simulink model "allInOne"  (R2018b)
settings: Solver=FixedStepDiscrete  StartTime=0.0  StopTime=inf  FixedStep=1/50  RelTol=1e-3  EnableMultiTasking=on
PreLoadFcn:
  | BOD_startup
  | BOW_startup
values from neighbouring files (symbols this model uses):
  K = Kext(1:6)    [BOW_startup.m]
  Rp = 4e-3    (= 0.004)    [BOW_startup.m]
undefined symbols (not defined in the file or in its folder): Ad, Ad1, Bd, Bd1, C, Cd, Dfilter, DiscIntNeverNeededParam, Discrete, F, G, K1, K2, K3, Kd, Ki, KN, Kp, KR, P_const, P_offset, sat, Time
libraries: simulink x4, ctrlSharedLib x4, embdlinuxlib x2
settings Model: SimulationMode=external  Creator=Josef  LastModifiedBy=Adam
settings SolverCC: PositivePriorityOrder=on
settings OptimizationCC: PassReuseOutputArgsThreshold=0  MaxStackSize=64
settings DebuggingCC: ParameterTunabilityLossMsg=error
settings HardwareCC: ProdBitPerPointer=32  ProdBitPerSizeT=32  ProdBitPerPtrDiffT=32  ProdLargestAtomicInteger=Long  ProdLargestAtomicFloat=Double  ProdWordSize=32  ProdHWDeviceType=ARM Compatible->ARM Cortex  UseEmbeddedCoderFeatures=off
settings SFSimCC: SimUseLocalCustomCode=off  MATLABDynamicMemAlloc=off
settings RTWCC: SystemTargetFile=ert.tlc  HardwareBoard=Raspberry Pi  TLCOptions="-aInlineSetEventsForThisBaseRateFcn=TLC_FALSE -aSuppressMultiTaskScheduler=TLC_FALSE  -aRateBasedStepFcn=0"  TemplateMakefile=ert_default_tmf  GenerateReport=on  RTWUseLocalCustomCode=off  Toolchain=GNU GCC Raspberry Pi  TargetLang=C++
settings CodeAppCC: ForceParamTrailComments=on  OperatorAnnotations=on  StateflowObjectComments=on
settings ERTTargetCC: TargetLangStandard=C++03 (ISO)  ERTCustomFileBanners=off  SupportContinuousTime=on  SupportNonInlinedSFcns=on  RemoveResetFunc=off  SupportVariableSizeSignals=on  ModelStepFunctionPrototypeControlCompliant=off

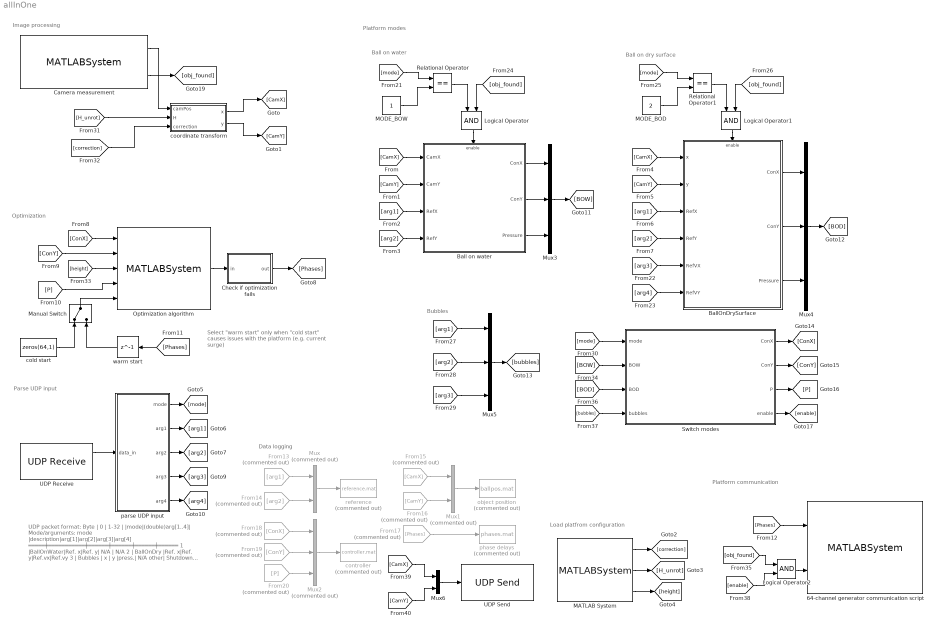
== system allInOne ==
  note: Platform modes
  note: UDP packet format:
      | Byte | 0 | 1-32 |
      | |mode|(double)arg[1..4]|
      |
      | Mode/arguments:
      | mode |description|arg[1]|arg[2]|arg[3]|arg[4]
      | ═════╪═══════════╪══════╪══════╪══════╪══════
      | 1 |BallOnWater|Ref. x|Ref. y| N/A | N/A
      | 2 | BallOnDry |Ref. x|Ref. y|Ref.vx|Ref.vy
      | 3 | Bubbles | x | y |press.| N/A
      | other| Shutdown | N/A | N/A | N/A | N/A
  note: Load platfrom configuration
  note: Select "warm start" only when
      | "cold start" causes issues with
      | the platform (e.g. current surge)
  note: Data logging
  note: Parse UDP input
  note: Platform communication
  note: Optimization
  note: Image processing
  note: Bubbles
  note: Ball on dry surface
  note: Ball on water
  64-channel generator communication script : MATLABSystem  System=NewGenerator  Port=/dev/ttyUSB0  Baud=230400
      mask Type: NewGenerator
      mask Display:
      | disp(['64 phase generator' char(10) ' Port: /dev/ttyUSB0' char(10) ' Baudrate: 230400']);
      | port_label('input',1,'phases');
      | port_label('input',2,'On/Off');
  Ball on water : Subsystem
  BallOnDrySurface : Subsystem
  Camera measurement : MATLABSystem  System=RaspiBallPos  shm_key=3145914  framerate=50  N=1000  objects=1  km=eye( 3 )  notfound=0  execScript=off  concatenateOutputs=off  rotation=off  found_output=on
      mask Type: RaspiBallPos
      mask Display:
      | disp('RaspiBallPos');
      | port_label('output',1,'Position 1 [x;y]');
      | port_label('output',2,'Object found?');
  Check if optimization fails : MATLAB Function  TreatAsAtomicUnit=on
  From13 : From  Commented=on  GotoTag=arg1
  From14 : From  Commented=on  GotoTag=arg2
  From15 : From  Commented=on  GotoTag=CamX
  From16 : From  Commented=on  GotoTag=CamY
  From17 : From  Commented=on  GotoTag=Phases
  From18 : From  Commented=on  GotoTag=ConX
  From19 : From  Commented=on  GotoTag=ConY
  From20 : From  Commented=on  GotoTag=P
  Logical Operator : Logic  AllPortsSameDT=off  OutDataTypeStr=boolean
  Logical Operator1 : Logic  AllPortsSameDT=off  OutDataTypeStr=boolean
  Logical Operator2 : Logic  AllPortsSameDT=off  OutDataTypeStr=boolean
  MATLAB System : MATLABSystem  System=Loader  corrFile=/home/pi/correction.bin  H_unFile=/home/pi/H_unrot.bin  heightFile=/home/pi/height.bin
      mask Type: Loader
      mask Display:
      | disp('Loader');
      | port_label('output',1,'correction');
      | port_label('output',2,'H_unrot');
      | port_label('output',3,'height');
  "MODE_BOD " : Constant  Value=2
  MODE_BOW : Constant
  Manual Switch : ManualSwitch
  Mux : Mux  Commented=on  Inputs=2
  Mux1 : Mux  Commented=on  Inputs=2
  Mux2 : Mux  Commented=on  Inputs=3
  Mux3 : Mux  Inputs=3
  Mux4 : Mux  Inputs=3
  Mux5 : Mux  Inputs=3
  Mux6 : Mux  Inputs=2
  Optimization algorithm : MATLABSystem  System=PressurePoints
      mask Type: PressurePoints
      mask Display:
      | disp(['Pressure points' char(10) 'optimization']);
      | port_label('input',1,'x');
      | port_label('input',2,'y');
      | port_label('input',3,'z');
      | port_label('input',4,'Required pressure');
      | port_label('input',5,'Initial condition');
      | port_label('output',1,'Phases');
  Relational Operator : RelationalOperator  Operator===  OutDataTypeStr=boolean  RndMeth=Simplest
  Relational Operator1 : RelationalOperator  Operator===  OutDataTypeStr=boolean  RndMeth=Simplest
  Switch modes : MATLAB Function  TreatAsAtomicUnit=on
  UDP Receive : embdlinuxlib/UDP Receive  localURL='0.0.0.0'  localPort=25000  remoteURL='0.0.0.0'  remotePort=-1  recvBufferSize=8192  signalDatatype=uint8  dims=33  isVarSize=off  showBlockingTime=off  blockingTime=0  sampletime=1/50  blockPlatform=Raspberry Pi
      settings: SourceProductName=Simulink Support Package for Raspberry Pi Hardware  SourceProductBaseCode=RASPPI
  UDP Send : embdlinuxlib/UDP Send  remoteURL='127.0.0.1'  remotePort=25001  localURL='255.255.255.255'  localPortSource=Automatically determine  localPort=-1  sampletime=-1  blockPlatform=Raspberry Pi  separateLengthPort=0
      settings: SourceProductName=Simulink Support Package for Raspberry Pi Hardware  SourceProductBaseCode=RASPPI
  cold start : Constant  Value=zeros(64,1)
  controller : ToFile  Commented=on  Filename=controller.mat  MatrixName=controller
  coordinate transform : MATLAB Function  TreatAsAtomicUnit=on
  object position : ToFile  Commented=on  Filename=ballpos.mat  MatrixName=ballpos
  parse UDP input : MATLAB Function  TreatAsAtomicUnit=on
  phase delays : ToFile  Commented=on  Filename=phases.mat  MatrixName=phases
  reference : ToFile  Commented=on  Filename=reference.mat  MatrixName=ref
  warm start : Delay  DelayLength=1  InitialCondition=zeros(64,1)
  wires:
  coordinate transform/1(x) -> [CamX]
  [H_unrot] -> coordinate transform/2(H)
  coordinate transform/2(y) -> [CamY]
  Camera measurement/1 -> coordinate transform/1(camPos)
  [correction] -> coordinate transform/3(correction)
  Check if optimization fails/1(out) -> [Phases]
  [ConX] -> Optimization algorithm/1
  [ConY] -> Optimization algorithm/2
  [Phases] -> warm start/1
  [P] -> Optimization algorithm/4
  Optimization algorithm/1 -> Check if optimization fails/1(in)
  cold start/1 -> Manual Switch/1
  warm start/1 -> Manual Switch/2
  Manual Switch/1 -> Optimization algorithm/5
  [height] -> Optimization algorithm/3
  [Phases] -> 64-channel generator communication script/1
  [obj_found] -> Logical Operator2/1
  From13/1 -> Mux/1
  From15/1 -> Mux1/1
  Mux1/1 -> object position/1
  From16/1 -> Mux1/2
  From18/1 -> Mux2/1
  From20/1 -> Mux2/3
  From19/1 -> Mux2/2
  Mux/1 -> reference/1
  From14/1 -> Mux/2
  From17/1 -> phase delays/1
  Mux2/1 -> controller/1
  MATLAB System/3 -> [height]
  MATLAB System/2 -> [H_unrot]
  MATLAB System/1 -> [correction]
  Camera measurement/2 -> [obj_found]
  UDP Receive/1 -> parse UDP input/1(data_in)
  parse UDP input/1(mode) -> [mode]
  parse UDP input/2(arg1) -> [arg1]
  parse UDP input/3(arg2) -> [arg2]
  parse UDP input/4(arg3) -> [arg3]
  parse UDP input/5(arg4) -> [arg4]
  [CamX] -> BallOnDrySurface/1(x)
  [arg1] -> BallOnDrySurface/3(RefX)
  Relational Operator/1 -> Logical Operator/1
  [arg2] -> BallOnDrySurface/4(RefY)
  [arg3] -> BallOnDrySurface/5(RefVX)
  MODE_BOW/1 -> Relational Operator/2
  Ball on water/2(ConY) -> Mux3/2
  [BOD] -> Switch modes/3(BOD)
  [CamY] -> BallOnDrySurface/2(y)
  [arg4] -> BallOnDrySurface/6(RefVY)
  BallOnDrySurface/2(ConY) -> Mux4/2
  BallOnDrySurface/1(ConX) -> Mux4/1
  [arg1] -> Mux5/1
  [arg2] -> Mux5/2
  [mode] -> Relational Operator/1
  BallOnDrySurface/3(Pressure) -> Mux4/3
  Mux5/1 -> [bubbles]
  Switch modes/3(P) -> [P]
  Ball on water/3(Pressure) -> Mux3/3
  [mode] -> Switch modes/1(mode)
  [CamY] -> Ball on water/2(CamY)
  Logical Operator/1 -> Ball on water/Enable
  "MODE_BOD "/1 -> Relational Operator1/2
  [mode] -> Relational Operator1/1
  [obj_found] -> Logical Operator1/2
  Logical Operator1/1 -> BallOnDrySurface/Enable
  Relational Operator1/1 -> Logical Operator1/1
  Mux3/1 -> [BOW]
  Switch modes/4(enable) -> [enable]
  Ball on water/1(ConX) -> Mux3/1
  [CamX] -> Ball on water/1(CamX)
  [arg2] -> Ball on water/4(RefY)
  [BOW] -> Switch modes/2(BOW)
  [arg1] -> Ball on water/3(RefX)
  [obj_found] -> Logical Operator/2
  [bubbles] -> Switch modes/4(bubbles)
  [arg3] -> Mux5/3
  Switch modes/1(ConX) -> [ConX]
  Switch modes/2(ConY) -> [ConY]
  Mux4/1 -> [BOD]
  Logical Operator2/1 -> 64-channel generator communication script/2
  [enable] -> Logical Operator2/2
  Mux6/1 -> UDP Send/1
  [CamX] -> Mux6/1
  [CamY] -> Mux6/2

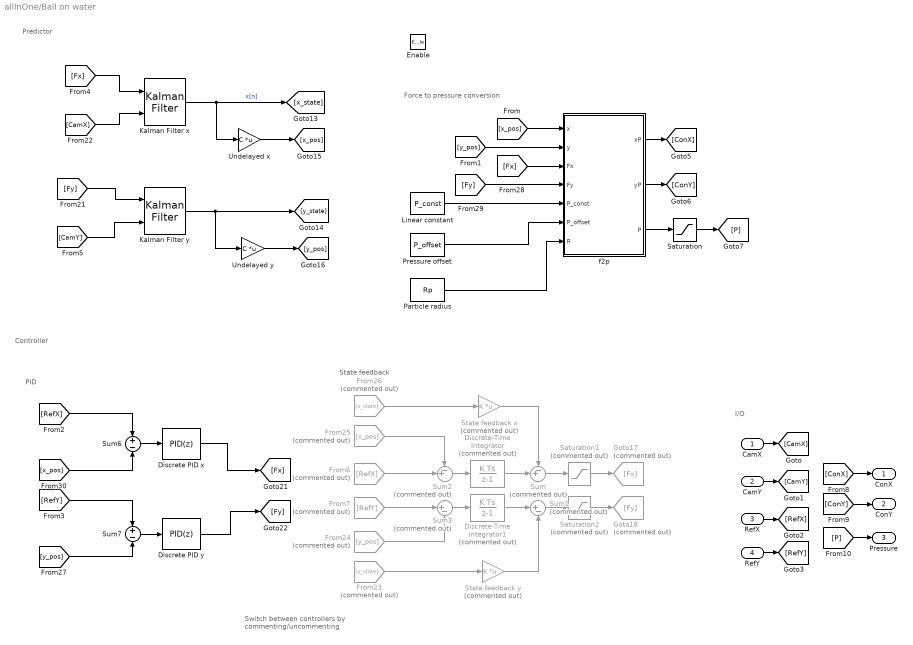
== system allInOne/Ball on water ==
  note: I/O
  note: Force to pressure conversion
  note: PID
  note: State feedback
  note: Switch between controllers by
      | commenting/uncommenting
  note: Controller
  note: Predictor
  CamX : Inport
  CamY : Inport  Port=2
  RefX : Inport  Port=3
  RefY : Inport  Port=4
  Enable : EnablePort  StatesWhenEnabling=reset
  Discrete PID x : simulink/Continuous/PID Controller  Controller=PID  Form=Parallel  TimeDomain=Discrete-time  SampleTime=-1  IntegratorMethod=Forward Euler  FilterMethod=Forward Euler  ControllerParametersSource=internal  P=Kp  I=Ki  D=Kd  UseFilter=on  N=Dfilter  TunerSelectOption=Transfer Function Based (PID Tuner App)  InitialConditionSource=internal  InitialConditionForIntegrator=0  InitialConditionForFilter=0  DifferentiatorICPrevScaledInput=0  ExternalReset=none  TrackingMode=off  Kt=1  LimitOutput=on  UpperSaturationLimit=sat  LowerSaturationLimit=-sat  LinearizeAsGain=off  AntiWindupMode=clamping  Kb=1  POutMin=[]  POutMax=[]  IOutMin=[]  IOutMax=[]  DOutMin=[]  DOutMax=[]  NOutMin=[]  NOutMax=[]  SumOutMin=[]  SumOutMax=[]  SaturationOutMin=[]  SaturationOutMax=[]  PParamMin=[]  PParamMax=[]  IParamMin=[]  IParamMax=[]  DParamMin=[]  DParamMax=[]  NParamMin=[]  NParamMax=[]  KbParamMin=[]  KbParamMax=[]  KtParamMin=[]  KtParamMax=[]  KbOutMin=[]  KbOutMax=[]  KtOutMin=[]  KtOutMax=[]  IntegratorOutMin=[]  IntegratorOutMax=[]  FilterOutMin=[]  FilterOutMax=[]  SumI1OutMin=[]  SumI1OutMax=[]  SumI2OutMin=[]  SumI2OutMax=[]  SumI3OutMin=[]  SumI3OutMax=[]  SumI4OutMin=[]  SumI4OutMax=[]  SumDOutMin=[]  SumDOutMax=[]  DifferentiatorOutMin=[]  DifferentiatorOutMax=[]  FilterDiffOutCoefMin=[]  FilterDiffOutCoefMax=[]  ReciprocalOutMin=[]  ReciprocalOutMax=[]  SumDenOutMin=[]  SumDenOutMax=[]  SumNumOutMin=[]  SumNumOutMax=[]  DivideOutMin=[]  DivideOutMax=[]  IntegratorContinuousStateAttributes=''  IntegratorStateMustResolveToSignalObject=off  IntegratorRTWStateStorageClass=Auto  FilterContinuousStateAttributes=''  FilterStateMustResolveToSignalObject=off  FilterRTWStateStorageClass=Auto  ParallelPVariant=InternalParameters  IdealPVariant=Disabled  IVariant=InternalParameters  DVariant=InternalParameters  IntegratorVariant=Discrete  SatVariant=Enabled  AWVariant=DiscClampingParallel  PCopyVariant=Disabled  TRVariant=Disabled  FdbkBlocksVariant=Forward  IdealPFdbkVariant=Disabled  SatFdbkVariant=Disabled  DerivativeFilterVariant=ForwardEulerFilter  NVariant=InternalParameters  NCopyVariant=Disabled  FilterICVariant=InternalICsFilter  IntegratorICVariant=InternalICs  ExternalResetVariant=Disabled  TRSumVariant=Passthrough  SumFdbkVariant=Disabled  SumVariant=Sum_PID
  Discrete PID y : simulink/Continuous/PID Controller  Controller=PID  Form=Parallel  TimeDomain=Discrete-time  SampleTime=-1  IntegratorMethod=Forward Euler  FilterMethod=Forward Euler  ControllerParametersSource=internal  P=Kp  I=Ki  D=Kd  UseFilter=on  N=Dfilter  TunerSelectOption=Frequency Response Based  InitialConditionSource=internal  InitialConditionForIntegrator=0  InitialConditionForFilter=0  DifferentiatorICPrevScaledInput=0  ExternalReset=none  TrackingMode=off  Kt=1  LimitOutput=on  UpperSaturationLimit=sat  LowerSaturationLimit=-sat  LinearizeAsGain=off  AntiWindupMode=clamping  Kb=1  POutMin=[]  POutMax=[]  IOutMin=[]  IOutMax=[]  DOutMin=[]  DOutMax=[]  NOutMin=[]  NOutMax=[]  SumOutMin=[]  SumOutMax=[]  SaturationOutMin=[]  SaturationOutMax=[]  PParamMin=[]  PParamMax=[]  IParamMin=[]  IParamMax=[]  DParamMin=[]  DParamMax=[]  NParamMin=[]  NParamMax=[]  KbParamMin=[]  KbParamMax=[]  KtParamMin=[]  KtParamMax=[]  KbOutMin=[]  KbOutMax=[]  KtOutMin=[]  KtOutMax=[]  IntegratorOutMin=[]  IntegratorOutMax=[]  FilterOutMin=[]  FilterOutMax=[]  SumI1OutMin=[]  SumI1OutMax=[]  SumI2OutMin=[]  SumI2OutMax=[]  SumI3OutMin=[]  SumI3OutMax=[]  SumI4OutMin=[]  SumI4OutMax=[]  SumDOutMin=[]  SumDOutMax=[]  DifferentiatorOutMin=[]  DifferentiatorOutMax=[]  FilterDiffOutCoefMin=[]  FilterDiffOutCoefMax=[]  ReciprocalOutMin=[]  ReciprocalOutMax=[]  SumDenOutMin=[]  SumDenOutMax=[]  SumNumOutMin=[]  SumNumOutMax=[]  DivideOutMin=[]  DivideOutMax=[]  IntegratorContinuousStateAttributes=''  IntegratorStateMustResolveToSignalObject=off  IntegratorRTWStateStorageClass=Auto  FilterContinuousStateAttributes=''  FilterStateMustResolveToSignalObject=off  FilterRTWStateStorageClass=Auto  ParallelPVariant=InternalParameters  IdealPVariant=Disabled  IVariant=InternalParameters  DVariant=InternalParameters  IntegratorVariant=Discrete  SatVariant=Enabled  AWVariant=DiscClampingParallel  PCopyVariant=Disabled  TRVariant=Disabled  FdbkBlocksVariant=Forward  IdealPFdbkVariant=Disabled  SatFdbkVariant=Disabled  DerivativeFilterVariant=ForwardEulerFilter  NVariant=InternalParameters  NCopyVariant=Disabled  FilterICVariant=InternalICsFilter  IntegratorICVariant=InternalICs  ExternalResetVariant=Disabled  TRSumVariant=Passthrough  SumFdbkVariant=Disabled  SumVariant=Sum_PID
  Discrete-Time Integrator : DiscreteIntegrator  Commented=on  gainval=K_i  SampleTime=1/50  UpperSaturationLimit=sat  LowerSaturationLimit=-sat  ICPrevOutput=DiscIntNeverNeededParam  ICPrevScaledInput=DiscIntNeverNeededParam
  Discrete-Time Integrator1 : DiscreteIntegrator  Commented=on  gainval=K_i  SampleTime=1/50  UpperSaturationLimit=sat  LowerSaturationLimit=-sat  ICPrevOutput=DiscIntNeverNeededParam  ICPrevScaledInput=DiscIntNeverNeededParam
  From23 : From  Commented=on  GotoTag=y_state
  From24 : From  Commented=on  GotoTag=y_pos
  From25 : From  Commented=on  GotoTag=x_pos
  From26 : From  Commented=on  GotoTag=x_state
  From6 : From  Commented=on  GotoTag=RefX
  From7 : From  Commented=on  GotoTag=RefY
  Goto17 : Goto  Commented=on  GotoTag=Fx
  Goto18 : Goto  Commented=on  GotoTag=Fy
  Kalman Filter x : ctrlSharedLib/Kalman Filter  TimeDomain=Discrete-Time  UseCurrentEstimator=on  ModelSource=Individual A, B, C, D matrices  ModelSourceVariable=ss(0.95,1,1,0,1)  A=F  B=G  C=C  D=0  NumberOfStates=1  NumberOfInputs=1  NumberOfOutputs=1  InitialEstimateSource=Dialog  X0=0  P0=10  UseK=off  UseGH=off  NumberOfProcessNoiseInputs=1  G=1  TimeInvariantG=on  H=0  TimeInvariantH=on  Q=KQ  TimeInvariantQ=on  R=KR  TimeInvariantR=on  N=KN  TimeInvariantN=on  AddInputPort=on  AddEnablePort=off  OutputEstimatedY=off  OutputP=off  Ts=1/50
      settings: SourceProductBaseCode=CT
  Kalman Filter y : ctrlSharedLib/Kalman Filter  TimeDomain=Discrete-Time  UseCurrentEstimator=on  ModelSource=Individual A, B, C, D matrices  ModelSourceVariable=ss(0.95,1,1,0,1)  A=F  B=G  C=C  D=0  NumberOfStates=1  NumberOfInputs=1  NumberOfOutputs=1  InitialEstimateSource=Dialog  X0=0  P0=10  UseK=off  UseGH=off  NumberOfProcessNoiseInputs=1  G=1  TimeInvariantG=on  H=0  TimeInvariantH=on  Q=KQ  TimeInvariantQ=on  R=KR  TimeInvariantR=on  N=KN  TimeInvariantN=on  AddInputPort=on  AddEnablePort=off  OutputEstimatedY=off  OutputP=off  Ts=1/50
      settings: SourceProductBaseCode=CT
  Linear constant : Constant  Value=P_const
  Particle radius : Constant  Value=Rp
  Pressure offset : Constant  Value=P_offset
  Saturation : Saturate  UpperLimit=2500  LowerLimit=0
  Saturation1 : Saturate  Commented=on  UpperLimit=sat  LowerLimit=-sat
  Saturation2 : Saturate  Commented=on  UpperLimit=sat  LowerLimit=-sat
  State feedback x : Gain  Commented=on  Gain=K  Multiplication=Matrix(K*u) (u vector)
  State feedback y : Gain  Commented=on  Gain=K  Multiplication=Matrix(K*u) (u vector)
  Sum : Sum  Commented=on  Inputs=-+|
  Sum1 : Sum  Commented=on  Inputs=|+-
  Sum2 : Sum  Commented=on  Inputs=-+|
  Sum3 : Sum  Commented=on  Inputs=|+-
  Sum6 : Sum  Inputs=+-
  Sum7 : Sum  Inputs=+-
  Undelayed x : Gain  Gain=C  Multiplication=Matrix(K*u)
  Undelayed y : Gain  Gain=C  Multiplication=Matrix(K*u)
  f2p : MATLAB Function  TreatAsAtomicUnit=on
  ConX : Outport
  ConY : Outport  Port=2
  Pressure : Outport  Port=3
  wires:
  [Fx] -> f2p/3(Fx)
  Pressure offset/1 -> f2p/6(P_offset)
  [x_pos] -> f2p/1(x)
  f2p/2(yP) -> [ConY]
  [Fy] -> f2p/4(Fy)
  Linear constant/1 -> f2p/5(P_const)
  Discrete PID x/1 -> [Fx]
  Discrete PID y/1 -> [Fy]
  f2p/3(P) -> Saturation/1
  [y_pos] -> f2p/2(y)
  Undelayed y/1 -> [y_pos]
  f2p/1(xP) -> [ConX]
  Saturation/1 -> [P]
  Particle radius/1 -> f2p/7(R)
  Undelayed x/1 -> [x_pos]
  Saturation2/1 -> Goto18/1
  Saturation1/1 -> Goto17/1
  Sum7/1 -> Discrete PID y/1
  [RefY] -> Sum7/1
  [y_pos] -> Sum7/2
  [x_pos] -> Sum6/2
  Sum6/1 -> Discrete PID x/1
  [RefX] -> Sum6/1
  [CamX] -> Kalman Filter x/2
  [Fx] -> Kalman Filter x/1
  Sum/1 -> Saturation1/1
  From26/1 -> State feedback x/1
  From7/1 -> Sum3/1
  From23/1 -> State feedback y/1
  From25/1 -> Sum2/1
  Sum1/1 -> Saturation2/1
  From24/1 -> Sum3/2
  From6/1 -> Sum2/2
  Sum3/1 -> Discrete-Time Integrator1/1
  State feedback x/1 -> Sum/1
  Sum2/1 -> Discrete-Time Integrator/1
  Discrete-Time Integrator/1 -> Sum/2
  Discrete-Time Integrator1/1 -> Sum1/1
  State feedback y/1 -> Sum1/2
  [ConX] -> ConX/1
  [ConY] -> ConY/1
  [P] -> Pressure/1
  CamX/1 -> [CamX]
  RefX/1 -> [RefX]
  CamY/1 -> [CamY]
  RefY/1 -> [RefY]
  [Fy] -> Kalman Filter y/1
  [CamY] -> Kalman Filter y/2
  Kalman Filter x/1 -> Undelayed x/1, [x_state]  "x[n]"
  Kalman Filter y/1 -> Undelayed y/1, [y_state]

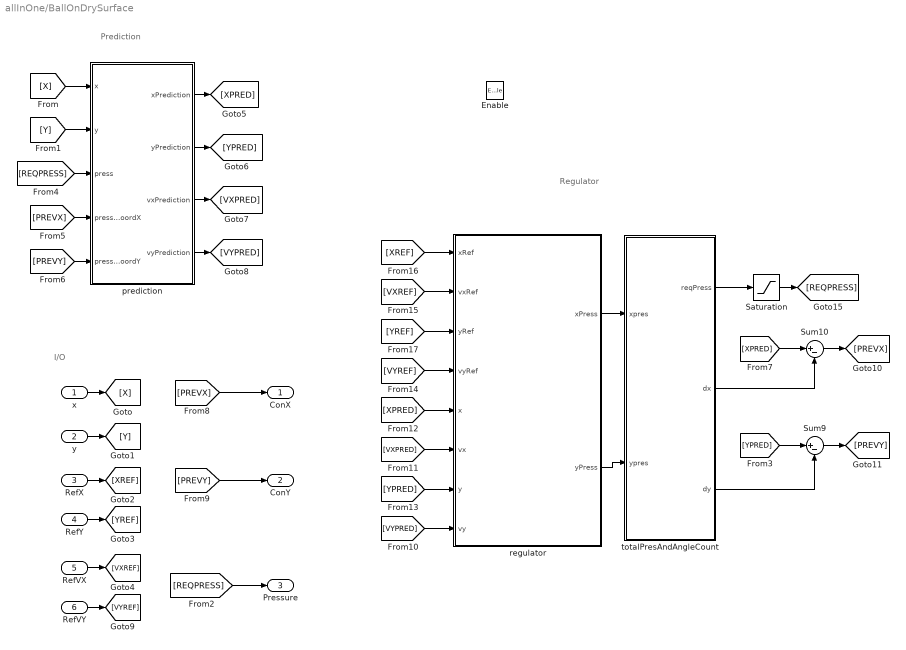
== system allInOne/BallOnDrySurface ==
  note: Prediction
  note: Regulator
  note: I/O
  x : Inport
  y : Inport  Port=2
  RefX : Inport  Port=3
  RefY : Inport  Port=4
  RefVX : Inport  Port=5
  RefVY : Inport  Port=6
  Enable : EnablePort  StatesWhenEnabling=reset
  Saturation : Saturate  UpperLimit=3300  LowerLimit=0
  Sum10 : Sum  Inputs=|+-
  Sum9 : Sum  Inputs=|+-
  prediction : Subsystem
  "regulator " : Subsystem
  totalPresAndAngleCount : MATLAB Function  TreatAsAtomicUnit=on
  ConX : Outport
  ConY : Outport  Port=2
  Pressure : Outport  Port=3
  wires:
  [X] -> prediction/1(x)
  prediction/4(vyPrediction) -> [VYPRED]
  prediction/3("vxPrediction ") -> [VXPRED]
  [REQPRESS] -> prediction/3("press ")
  [Y] -> prediction/2(y)
  prediction/2(yPrediction) -> [YPRED]
  prediction/1(xPrediction) -> [XPRED]
  [PREVY] -> prediction/5("pressCoordY ")
  [PREVX] -> prediction/4(pressCoordX)
  [XPRED] -> "regulator "/5(x)
  [VXREF] -> "regulator "/2(vxRef)
  [VXPRED] -> "regulator "/6(vx)
  [YPRED] -> "regulator "/7(y)
  [XREF] -> "regulator "/1(xRef)
  Saturation/1 -> [REQPRESS]
  [YREF] -> "regulator "/3(yRef)
  "regulator "/2(yPress) -> totalPresAndAngleCount/2(ypres)
  "regulator "/1(xPress) -> totalPresAndAngleCount/1(xpres)
  totalPresAndAngleCount/1(reqPress) -> Saturation/1
  [VYREF] -> "regulator "/4(vyRef)
  [VYPRED] -> "regulator "/8(vy)
  x/1 -> [X]
  Sum10/1 -> [PREVX]
  y/1 -> [Y]
  RefX/1 -> [XREF]
  Sum9/1 -> [PREVY]
  RefY/1 -> [YREF]
  [REQPRESS] -> Pressure/1
  RefVY/1 -> [VYREF]
  RefVX/1 -> [VXREF]
  [YPRED] -> Sum9/1
  [XPRED] -> Sum10/1
  totalPresAndAngleCount/2(dx) -> Sum10/2
  totalPresAndAngleCount/3(dy) -> Sum9/2
  [PREVX] -> ConX/1
  [PREVY] -> ConY/1

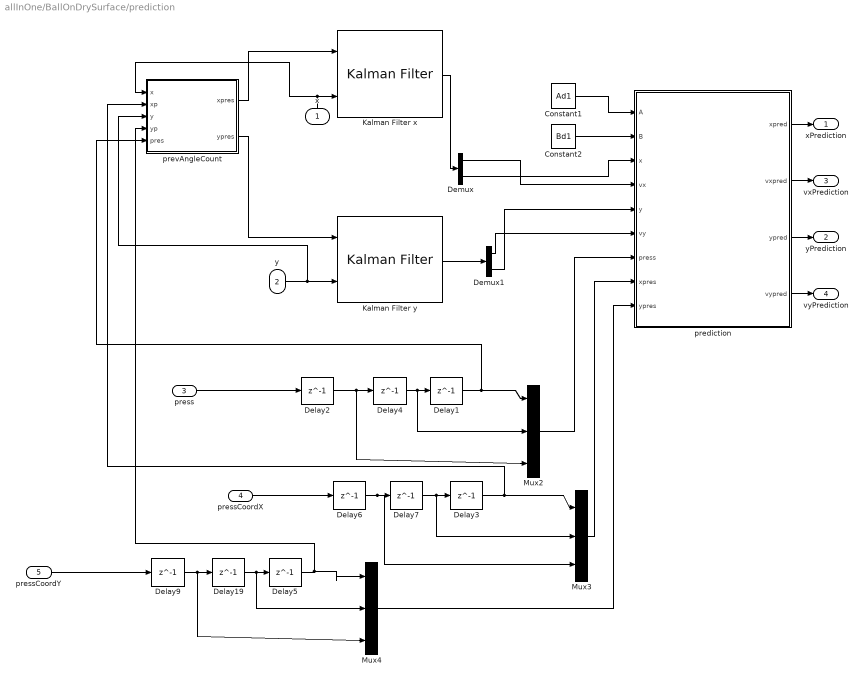
== system allInOne/BallOnDrySurface/prediction ==
  x : Inport  SampleTime=1/50
  y : Inport  Port=2  SampleTime=1/50
  "press " : Inport  Port=3
  pressCoordX : Inport  Port=4
  "pressCoordY " : Inport  Port=5
  Constant1 : Constant  Value=Ad1  SampleTime=-1
  Constant2 : Constant  Value=Bd1  SampleTime=-1
  Delay{1..7,9,19} (9 alike) : Delay  DelayLength=1
  Demux : Demux  Outputs=2
  Demux1 : Demux  Outputs=2
  Kalman Filter x : ctrlSharedLib/Kalman Filter  TimeDomain=Discrete-Time  UseCurrentEstimator=on  ModelSource=Individual A, B, C, D matrices  ModelSourceVariable=ss(0.95,1,1,0,1)  A=Ad  B=Bd  C=Cd  D=0  NumberOfStates=1  NumberOfInputs=1  NumberOfOutputs=1  InitialEstimateSource=Dialog  X0=[0;0]  P0=10  UseK=off  UseGH=off  NumberOfProcessNoiseInputs=1  G=1  TimeInvariantG=on  H=0  TimeInvariantH=on  Q=[5e-5 0 ; 0 1e-7]  TimeInvariantQ=on  R=7e-12;  TimeInvariantR=on  N=0  TimeInvariantN=on  AddInputPort=on  AddEnablePort=off  OutputEstimatedY=off  OutputP=off  Ts=-1
      settings: SourceProductBaseCode=CT
  Kalman Filter y : ctrlSharedLib/Kalman Filter  TimeDomain=Discrete-Time  UseCurrentEstimator=on  ModelSource=Individual A, B, C, D matrices  ModelSourceVariable=ss(0.95,1,1,0,1)  A=Ad  B=Bd  C=Cd  D=0  NumberOfStates=1  NumberOfInputs=1  NumberOfOutputs=1  InitialEstimateSource=Dialog  X0=[0;0]  P0=10  UseK=off  UseGH=off  NumberOfProcessNoiseInputs=1  G=1  TimeInvariantG=on  H=0  TimeInvariantH=on  Q=[5e-5 0 ; 0 1e-7]  TimeInvariantQ=on  R=7e-12;  TimeInvariantR=on  N=0  TimeInvariantN=on  AddInputPort=on  AddEnablePort=off  OutputEstimatedY=off  OutputP=off  Ts=-1
      settings: SourceProductBaseCode=CT
  Mux2 : Mux  Inputs=3
  Mux3 : Mux  Inputs=3
  Mux4 : Mux  Inputs=3
  prediction : MATLAB Function  TreatAsAtomicUnit=on
  prevAngleCount : MATLAB Function  TreatAsAtomicUnit=on
  xPrediction : Outport
  yPrediction : Outport  Port=2
  "vxPrediction " : Outport  Port=3
  vyPrediction : Outport  Port=4
  wires:
  prediction/1(xpred) -> xPrediction/1
  prediction/3(ypred) -> yPrediction/1
  prediction/2(vxpred) -> "vxPrediction "/1
  prediction/4(vypred) -> vyPrediction/1
  Constant2/1 -> prediction/2(B)
  Constant1/1 -> prediction/1(A)
  x/1 -> prevAngleCount/1(x), Kalman Filter x/2
  y/1 -> prevAngleCount/3(y), Kalman Filter y/2
  Delay4/1 -> Mux2/2, Delay1/1
  Mux2/1 -> prediction/7(press)
  Delay7/1 -> Mux3/2, Delay3/1
  Delay19/1 -> Mux4/2, Delay5/1
  Mux3/1 -> prediction/8(xpres)
  Mux4/1 -> prediction/9(ypres)
  prevAngleCount/1(xpres) -> Kalman Filter x/1
  Kalman Filter x/1 -> Demux/1
  Demux/1 -> prediction/4(vx)
  prevAngleCount/2(ypres) -> Kalman Filter y/1
  Kalman Filter y/1 -> Demux1/1
  Demux1/1 -> prediction/6(vy)
  Demux/2 -> prediction/3(x)
  Demux1/2 -> prediction/5(y)
  Delay2/1 -> Mux2/3, Delay4/1
  Delay6/1 -> Mux3/3, Delay7/1
  Delay9/1 -> Mux4/3, Delay19/1
  "pressCoordY "/1 -> Delay9/1
  pressCoordX/1 -> Delay6/1
  "press "/1 -> Delay2/1
  Delay1/1 -> prevAngleCount/5(pres), Mux2/1
  Delay3/1 -> prevAngleCount/2(xp), Mux3/1
  Delay5/1 -> Mux4/1, prevAngleCount/4(yp)

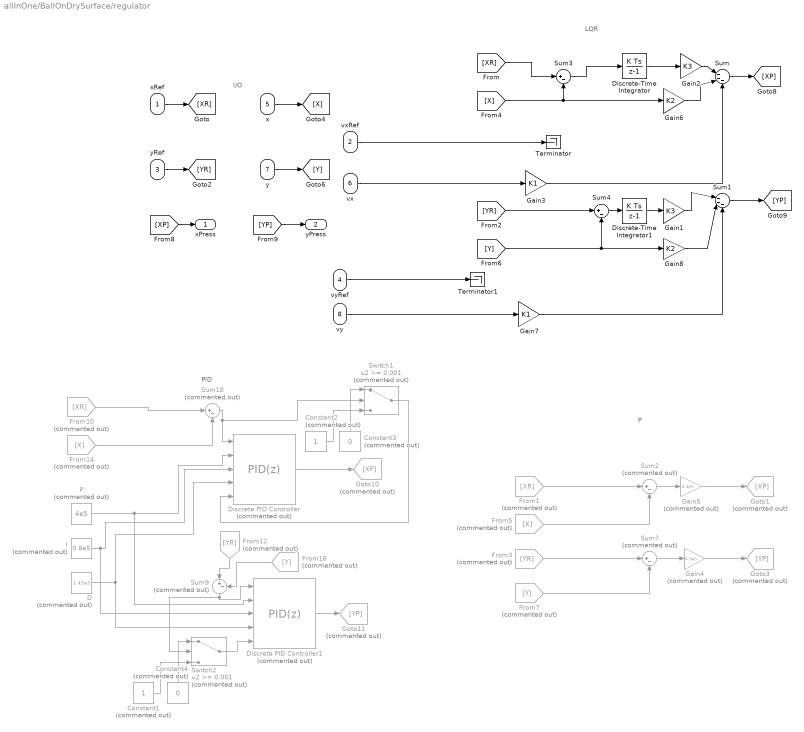
== system allInOne/BallOnDrySurface/regulator  ==
  note: P
  note: I/O
  note: LQR
  note: PID
  xRef : Inport
  vxRef : Inport  Port=2
  yRef : Inport  Port=3
  vyRef : Inport  Port=4
  x : Inport  Port=5
  vx : Inport  Port=6
  y : Inport  Port=7
  vy : Inport  Port=8
  Constant1 : Constant  Commented=on
  Constant2 : Constant  Commented=on
  Constant3 : Constant  Commented=on  Value=0
  Constant4 : Constant  Commented=on  Value=0
  D : Constant  Commented=on  Value=1.45e5
  Discrete PID Controller : simulink/Continuous/PID Controller  Commented=on  Controller=PID  Form=Parallel  TimeDomain=Discrete-time  SampleTime=-1  IntegratorMethod=Forward Euler  FilterMethod=Forward Euler  ControllerParametersSource=external  P=14.5e5  I=0.8e5  D=2e5  UseFilter=off  N=95.4163407177024  TunerSelectOption=Transfer Function Based (PID Tuner App)  InitialConditionSource=internal  InitialConditionForIntegrator=0  InitialConditionForFilter=0  DifferentiatorICPrevScaledInput=0  ExternalReset=rising  TrackingMode=off  Kt=1  LimitOutput=on  UpperSaturationLimit=3300  LowerSaturationLimit=-3300  LinearizeAsGain=off  AntiWindupMode=clamping  Kb=1  POutMin=[]  POutMax=[]  IOutMin=[]  IOutMax=[]  DOutMin=[]  DOutMax=[]  NOutMin=[]  NOutMax=[]  SumOutMin=[]  SumOutMax=[]  SaturationOutMin=[]  SaturationOutMax=[]  PParamMin=[]  PParamMax=[]  IParamMin=[]  IParamMax=[]  DParamMin=[]  DParamMax=[]  NParamMin=[]  NParamMax=[]  KbParamMin=[]  KbParamMax=[]  KtParamMin=[]  KtParamMax=[]  KbOutMin=[]  KbOutMax=[]  KtOutMin=[]  KtOutMax=[]  IntegratorOutMin=[]  IntegratorOutMax=[]  FilterOutMin=[]  FilterOutMax=[]  SumI1OutMin=[]  SumI1OutMax=[]  SumI2OutMin=[]  SumI2OutMax=[]  SumI3OutMin=[]  SumI3OutMax=[]  SumI4OutMin=[]  SumI4OutMax=[]  SumDOutMin=[]  SumDOutMax=[]  DifferentiatorOutMin=[]  DifferentiatorOutMax=[]  FilterDiffOutCoefMin=[]  FilterDiffOutCoefMax=[]  ReciprocalOutMin=[]  ReciprocalOutMax=[]  SumDenOutMin=[]  SumDenOutMax=[]  SumNumOutMin=[]  SumNumOutMax=[]  DivideOutMin=[]  DivideOutMax=[]  IntegratorContinuousStateAttributes=''  IntegratorStateMustResolveToSignalObject=off  IntegratorRTWStateStorageClass=Auto  FilterContinuousStateAttributes=''  FilterStateMustResolveToSignalObject=off  FilterRTWStateStorageClass=Auto  ParallelPVariant=ExternalParameters  IdealPVariant=Disabled  IVariant=ExternalParameters  DVariant=ExternalParameters  IntegratorVariant=Discrete  SatVariant=Enabled  AWVariant=DiscClampingParallel  PCopyVariant=Disabled  TRVariant=Disabled  FdbkBlocksVariant=Forward  IdealPFdbkVariant=Disabled  SatFdbkVariant=Disabled  DerivativeFilterVariant=Differentiator  NVariant=Passthrough  NCopyVariant=Disabled_SignalSpec  FilterICVariant=InternalICsDifferentiator  IntegratorICVariant=InternalICs  ExternalResetVariant=ExternalReset  TRSumVariant=Passthrough  SumFdbkVariant=Disabled  SumVariant=Sum_PID
  Discrete PID Controller1 : simulink/Continuous/PID Controller  Commented=on  Controller=PID  Form=Parallel  TimeDomain=Discrete-time  SampleTime=-1  IntegratorMethod=Forward Euler  FilterMethod=Forward Euler  ControllerParametersSource=external  P=14.5e5  I=0.8e5  D=2e5  UseFilter=off  N=95.4163407177024  TunerSelectOption=Transfer Function Based (PID Tuner App)  InitialConditionSource=internal  InitialConditionForIntegrator=0  InitialConditionForFilter=0  DifferentiatorICPrevScaledInput=0  ExternalReset=rising  TrackingMode=off  Kt=1  LimitOutput=on  UpperSaturationLimit=3300  LowerSaturationLimit=-3300  LinearizeAsGain=off  AntiWindupMode=clamping  Kb=1  POutMin=[]  POutMax=[]  IOutMin=[]  IOutMax=[]  DOutMin=[]  DOutMax=[]  NOutMin=[]  NOutMax=[]  SumOutMin=[]  SumOutMax=[]  SaturationOutMin=[]  SaturationOutMax=[]  PParamMin=[]  PParamMax=[]  IParamMin=[]  IParamMax=[]  DParamMin=[]  DParamMax=[]  NParamMin=[]  NParamMax=[]  KbParamMin=[]  KbParamMax=[]  KtParamMin=[]  KtParamMax=[]  KbOutMin=[]  KbOutMax=[]  KtOutMin=[]  KtOutMax=[]  IntegratorOutMin=[]  IntegratorOutMax=[]  FilterOutMin=[]  FilterOutMax=[]  SumI1OutMin=[]  SumI1OutMax=[]  SumI2OutMin=[]  SumI2OutMax=[]  SumI3OutMin=[]  SumI3OutMax=[]  SumI4OutMin=[]  SumI4OutMax=[]  SumDOutMin=[]  SumDOutMax=[]  DifferentiatorOutMin=[]  DifferentiatorOutMax=[]  FilterDiffOutCoefMin=[]  FilterDiffOutCoefMax=[]  ReciprocalOutMin=[]  ReciprocalOutMax=[]  SumDenOutMin=[]  SumDenOutMax=[]  SumNumOutMin=[]  SumNumOutMax=[]  DivideOutMin=[]  DivideOutMax=[]  IntegratorContinuousStateAttributes=''  IntegratorStateMustResolveToSignalObject=off  IntegratorRTWStateStorageClass=Auto  FilterContinuousStateAttributes=''  FilterStateMustResolveToSignalObject=off  FilterRTWStateStorageClass=Auto  ParallelPVariant=ExternalParameters  IdealPVariant=Disabled  IVariant=ExternalParameters  DVariant=ExternalParameters  IntegratorVariant=Discrete  SatVariant=Enabled  AWVariant=DiscClampingParallel  PCopyVariant=Disabled  TRVariant=Disabled  FdbkBlocksVariant=Forward  IdealPFdbkVariant=Disabled  SatFdbkVariant=Disabled  DerivativeFilterVariant=Differentiator  NVariant=Passthrough  NCopyVariant=Disabled_SignalSpec  FilterICVariant=InternalICsDifferentiator  IntegratorICVariant=InternalICs  ExternalResetVariant=ExternalReset  TRSumVariant=Passthrough  SumFdbkVariant=Disabled  SumVariant=Sum_PID  InitialConditionSetting=Output
  Discrete-Time Integrator : DiscreteIntegrator  gainval=1  SampleTime=-1  ICPrevOutput=DiscIntNeverNeededParam  ICPrevScaledInput=DiscIntNeverNeededParam
  Discrete-Time Integrator1 : DiscreteIntegrator  gainval=1  SampleTime=-1  ICPrevOutput=DiscIntNeverNeededParam  ICPrevScaledInput=DiscIntNeverNeededParam
  From1 : From  Commented=on  GotoTag=XR
  From10 : From  Commented=on  GotoTag=XR
  From12 : From  Commented=on  GotoTag=YR
  From14 : From  Commented=on  GotoTag=X
  From16 : From  Commented=on  GotoTag=Y
  From3 : From  Commented=on  GotoTag=YR
  From5 : From  Commented=on  GotoTag=X
  From7 : From  Commented=on  GotoTag=Y
  Gain1 : Gain  Gain=K3
  Gain2 : Gain  Gain=K3
  Gain3 : Gain  Gain=K1
  Gain4 : Gain  Commented=on  Gain=4.3e5
  Gain5 : Gain  Commented=on  Gain=4.3e5
  Gain6 : Gain  Gain=K2
  Gain7 : Gain  Gain=K1
  Gain8 : Gain  Gain=K2
  Goto1 : Goto  Commented=on  GotoTag=XP
  Goto10 : Goto  Commented=on  GotoTag=XP
  Goto11 : Goto  Commented=on  GotoTag=YP
  Goto3 : Goto  Commented=on  GotoTag=YP
  I : Constant  Commented=on  Value=0.8e5
  P : Constant  Commented=on  Value=4e5
  Sum : Sum  Inputs=|---
  Sum1 : Sum  Inputs=|---
  Sum{2,7,9..10} (4 alike) : Sum  Commented=on  Inputs=|+-
  Sum3 : Sum  Inputs=|+-
  Sum4 : Sum  Inputs=|+-
  Switch1 : Switch  Commented=on  Threshold=0.001
  Switch2 : Switch  Commented=on  Threshold=0.001
  Terminator : Terminator
  Terminator1 : Terminator
  xPress : Outport
  yPress : Outport  Port=2
  wires:
  xRef/1 -> [XR]
  yRef/1 -> [YR]
  x/1 -> [X]
  y/1 -> [Y]
  [XR] -> Sum3/1
  [YR] -> Sum4/1
  vxRef/1 -> Terminator/1
  [X] -> Sum3/2, Gain6/1
  vx/1 -> Gain3/1
  [Y] -> Sum4/2, Gain8/1
  vy/1 -> Gain7/1
  Sum/1 -> [XP]
  Sum1/1 -> [YP]
  [XP] -> xPress/1
  [YP] -> yPress/1
  Discrete PID Controller/1 -> Goto10/1
  From16/1 -> Sum9/2
  From12/1 -> Sum9/1
  Discrete PID Controller1/1 -> Goto11/1
  From14/1 -> Sum10/2
  From10/1 -> Sum10/1
  Sum10/1 -> Switch1/2, Discrete PID Controller/1
  Sum9/1 -> Switch2/2, Discrete PID Controller1/1
  P/1 -> Discrete PID Controller1/2, Discrete PID Controller/2
  I/1 -> Discrete PID Controller1/3, Discrete PID Controller/3
  D/1 -> Discrete PID Controller1/4, Discrete PID Controller/4
  Gain5/1 -> Goto1/1
  Sum2/1 -> Gain5/1
  Sum7/1 -> Gain4/1
  From7/1 -> Sum7/2
  Gain4/1 -> Goto3/1
  From1/1 -> Sum2/1
  From3/1 -> Sum7/1
  From5/1 -> Sum2/2
  Constant2/1 -> Switch1/3
  Constant3/1 -> Switch1/1
  Constant4/1 -> Switch2/1
  Constant1/1 -> Switch2/3
  Switch2/1 -> Discrete PID Controller1/5
  Switch1/1 -> Discrete PID Controller/5
  Gain7/1 -> Sum1/3
  Gain3/1 -> Sum/3
  Gain6/1 -> Sum/2
  Sum3/1 -> Discrete-Time Integrator/1
  Discrete-Time Integrator/1 -> Gain2/1
  vyRef/1 -> Terminator1/1
  Gain8/1 -> Sum1/2
  Sum4/1 -> Discrete-Time Integrator1/1
  Discrete-Time Integrator1/1 -> Gain1/1
  Gain1/1 -> Sum1/1
  Gain2/1 -> Sum/1

== matlab function allInOne/coordinate transform ==
  data: x output; camPos input; y output; H input; correction input
function [x,y] = trans(camPos, H, correction)
    [x,y] = coordTransform(H, camPos, correction);
end

== matlab function allInOne/BallOnDrySurface/prediction/prevAngleCount ==
  data: x input; xpres output; xp input; y input; yp input; pres input; ypres output
function [xpres,ypres] = prevAngleCount(x,xp,y,yp, pres)
angl = atan2((y-yp),(x-xp));
xpres = pres*cos(angl);
ypres = pres*sin(angl);

== matlab function allInOne/Check if optimization fails ==
  data: in input; out output
function out = NaNcontrol(in)
    if isnan(in)
        out = zeros(64,1);
    else
        out = in;
    end
% % end

== matlab function allInOne/Ball on water/f2p ==
  data: x input; xP output; y input; Fx input; Fy input; P_const input; P_offset input; R input; yP output; P output
function [xP,yP,P] = forceToPressure(x,y,Fx,Fy,P_const,P_offset,R)    
    F = sqrt(Fx^2 + Fy^2);
    P = P_const*F + P_offset;
    cosA = Fx/F;
    sinA = Fy/F;
    xP = x - (R+0.0015)*cosA;
    yP = y - (R+0.0015)*sinA;
end

== matlab function allInOne/BallOnDrySurface/prediction/prediction ==
  data: A input; B input; x input; vx input; y input; vy input; press input; xpres input; ypres input; xpred output; vxpred output; ypred output; vypred output
function [xpred, vxpred,ypred,vypred] = prediction(A,B,x,vx,y,vy,press,xpres, ypres)

delay = 3;
 ux = zeros(delay,1);
 uy = zeros(delay,1);
 angle = zeros(delay,1);
 angle(1) = atan2(y-ypres(1),x-xpres(1));
 ux(1) = cos(angle(1))*press(1);
 uy(1) = sin(angle(1))*press(1);
 z = [vx;x;vy;y];
for i =1:delay
z = A*z + B*[ux(i);uy(i)];
 if i < delay
 angle(i+1) = atan2(z(4)-ypres(i+1),z(2)-xpres(i+1));
 ux(i+1) = cos(angle(i+1))*press(i+1);
 uy(i+1) = sin(angle(i+1))*press(i+1);
 end
end
 vxpred = z(1);
 xpred = z(2);
 vypred = z(3);
 ypred = z(4);

== matlab function allInOne/BallOnDrySurface/totalPresAndAngleCount ==
  data: xpres input; ypres input; reqPress output; dx output; dy output
function [reqPress,dx,dy] = totalPresAndAngleCount(xpres,ypres)
reqPress = sqrt(xpres^2+ypres^2);
alpha = atan2(ypres,xpres);
dx = 0.003*cos(alpha);
dy = 0.003*sin(alpha);

== matlab function allInOne/parse UDP input ==
  data: data_in input; mode output; arg1 output; arg2 output; arg3 output; arg4 output
function [mode,arg1,arg2,arg3,arg4] = parseInput(data_in)
    mode = data_in(1);
    args = typecast(data_in(2:end),'double');
    arg1 = args(1);
    arg2 = args(2);
    arg3 = args(3);
    arg4 = args(4);

== matlab function allInOne/Switch modes ==
  data: mode input; ConX output; BOW input; BOD input; bubbles input; ConY output; P output; enable output
function [ConX,ConY,P,enable] = switcher(mode,BOW,BOD,bubbles)
    switch mode
        case 1
            ConX = BOW(1);
            ConY = BOW(2);
            P = BOW(3);
            enable = true;
        case 2
            ConX = BOD(1);
            ConY = BOD(2);
            P = BOD(3);
            enable = true;
        case 3
            ConX = bubbles(1);
            ConY = bubbles(2);
            P = bubbles(3);
            enable = true;
        otherwise
            ConX = 0;
            ConY = 0;
            P = 0;
            enable = false;
    end
